simulink model "test"  (Simulink 7.4)
settings: Solver=ode45  StartTime=0.0  StopTime=100  MaxStep=0.05  RelTol=1e-3
values from neighbouring files (symbols this model uses):
  n_delay = [0; 40]    [setup.m]
  P_D = x(end)    [comp_rig_parallel_linearized.m]    (also in comp_rig_tank.m = x(1); get_tank_deriv.m = x(1); setup.m = xinit(end); test_linearization.m = P_D_init + delta_x(end,i))
  Ts = 0.05    [const_sim.m]
  uoff1 = [0.304, 0.405, 0.393, 0]'    [const_sim.m]
  uoff2 = [0.304, 0.405, 0.393, 0]'    [const_sim.m]
  xinit = [ 0.87171 1.0425 0.17319 400.38      0 0.98528 1.1784 0.17319 400.38      0 1.0116 ]    [setup.m]    (also in test_linearization.m = [0.890; 1.096; 0.159; 426; 0)
settings Model: Creator=chkajon  LastModifiedBy=chkajon

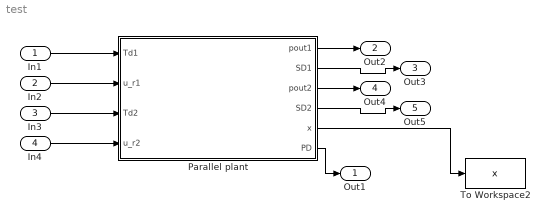
== system test ==
  In1 : Inport  OutDataType=fixdt(1, 16)  OutScaling=2^0
  In2 : Inport  Port=2  OutDataType=fixdt(1, 16)  OutScaling=2^0
  In3 : Inport  Port=3  OutDataType=fixdt(1, 16)  OutScaling=2^0
  In4 : Inport  Port=4  OutDataType=fixdt(1, 16)  OutScaling=2^0
  Parallel plant : Subsystem  mask{x_init_total=xinit, disturbances_on=off, disturbances_symm=off, dist_t_in=0, dist1_in=0, dist2_in=0}
      mask prompts: x_init_total "Initial state"; disturbances_on "Activate disturbances"; disturbances_symm "Symmetric disturbances"; dist_t_in "Disturbance times (up to 2)"; dist1_in "Disturbance 1 values (u1in, u1out, ud[, u2in, u2out])"; dist2_in "Disturbance 2 values"
      mask init:
      | dist1 = zeros(5,1);
      | dist2 = dist1;
      | dist_t = zeros(2,1);
      | 
      | if disturbances_on
      |     for i=1:min(5,length(dist1_in))
      |         dist1(i) = dist1_in(i);
      |     end
      |     for i=1:min(5,length(dist2_in))
      |         dist2(i) = dist2_in(i);
      |     end
      |     for i=1:min(2,length(dist_t_in))
      |         dist_t(i) = dist_t_in(i);
      |     end
      |     
      |     if disturbances_symm
      |         dist1(4) = dist1(1);
      |         dist1(5) = dist1(2);
      |         dist2(4) = dist2(1);
      |         dist2(5) = dist2(2);
      |     end
      | end
      | 
      | x_init1 = x_init_total(1:5);
      | x_init2 = x_init_total(6:10);
  To Workspace2 : ToWorkspace  VariableName=x  SampleTime=-1  SaveFormat=Structure With Time
  Out1 : Outport  OutDataType=fixdt(1, 16)  OutScaling=2^0
  Out2 : Outport  Port=2  OutDataType=fixdt(1, 16)  OutScaling=2^0
  Out3 : Outport  Port=3  OutDataType=fixdt(1, 16)  OutScaling=2^0
  Out4 : Outport  Port=4  OutDataType=fixdt(1, 16)  OutScaling=2^0
  Out5 : Outport  Port=5  OutDataType=fixdt(1, 16)  OutScaling=2^0
  wires:
  In1/1 -> Parallel plant/1(Td1)
  In2/1 -> Parallel plant/2(u_r1)
  In3/1 -> Parallel plant/3(Td2)
  In4/1 -> Parallel plant/4(u_r2)
  Parallel plant/5(x) -> To Workspace2/1
  Parallel plant/6(PD) -> Out1/1
  Parallel plant/1(pout1) -> Out2/1
  Parallel plant/2(SD1) -> Out3/1
  Parallel plant/3(pout2) -> Out4/1
  Parallel plant/4(SD2) -> Out5/1

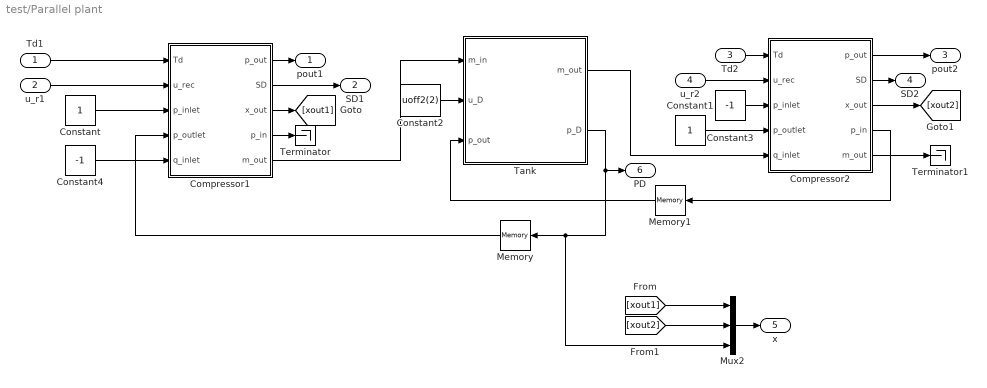
== system test/Parallel plant ==
  Td1 : Inport  OutDataType=fixdt(1, 16)  OutScaling=2^0
  u_r1 : Inport  Port=2  OutDataType=fixdt(1, 16)  OutScaling=2^0
  Td2 : Inport  Port=3  OutDataType=fixdt(1, 16)  OutScaling=2^0
  u_r2 : Inport  Port=4  OutDataType=fixdt(1, 16)  OutScaling=2^0
  Compressor1 : Subsystem  mask(Compressor){x_init=x_init1, Td_off=uoff1(1), u_in=uoff1(2), u_out=uoff1(3), u_rec=uoff1(4), t_delay=n_delay(2)*Ts, use_dist=on, u_out_dist=[dist1(1); dist2(1)], u_out_time=dist_t, u_in_dist=[dist1(2); dist2(2)], u_in_time=dist_t}
      mask prompts: x_init "Intial state"; Td_off "Torque offset"; u_in "Input valve setting"; u_out "Output valve setting"; u_rec "Recycle valve offset"; t_delay "Recycle valve time delay"; use_dist "Activate valve disturbances"; u_out_dist "Output valve disturbance magnitudes (up to 2)"; u_out_time "Output valve disturbance times (up to 2)"; u_in_dist "Input valve disturbance magnitudes (up to 2)"; u_in_time "Input valve disturbance times (up to 2)"
      mask help: Compressor with tunable inputs.
      mask init:
      | if use_dist
      |     n = min(length(u_out_dist),length(u_out_time));
      |     if n==0
      |         u_out_dist = [0;0];
      |         u_out_time = [0;0];
      |     elseif n==1
      |         u_out_dist = [u_out_dist(1);0];
      |         u_out_time = [u_out_time(1);0];
      |     else
      |         u_out_dist = [u_out_dist(1);u_out_dist(2)];
      |         u_out_time = [u_out_time(1); u_out_time(2)];
      |     end
      |     
      |     n = min(length(u_in_dist),length(u_in_time));
      |     if n==0
      |         u_in_dist = [0;0];
      |         u_in_time = [0;0];
      |     elseif n==1
      |         u_in_dist = [u_in_dist(1);0];
      |         u_in_time = [u_in_time(1);0];
      |     else
      |         u_in_dist = [u_in_dist(1);u_in_dist(2)];
      |         u_in_time = [u_in_time(1); u_in_time(2)];
      |     end
      | else
      |     u_out_dist = [0;0];
      |     u_out_time = [0;0];
      |     u_in_dist = [0;0];
      |     u_in_time = [0;0];
      | end
      mask TabNameString: Disturbances,Inputs,Inputs,Inputs,Inputs,Inputs,Disturbances,Disturbances,Disturbances,Disturbances,Disturbances
  Compressor2 : Subsystem  mask(Compressor){x_init=x_init2, Td_off=uoff2(1), u_in=uoff2(2), u_out=uoff2(3), u_rec=uoff2(4), t_delay=n_delay(2)*Ts, use_dist=on, u_out_dist=[dist1(4); dist2(4)], u_out_time=dist_t, u_in_dist=[dist1(5); dist2(5)], u_in_time=dist_t}
      mask prompts: x_init "Intial state"; Td_off "Torque offset"; u_in "Input valve setting"; u_out "Output valve setting"; u_rec "Recycle valve offset"; t_delay "Recycle valve time delay"; use_dist "Activate valve disturbances"; u_out_dist "Output valve disturbance magnitudes (up to 2)"; u_out_time "Output valve disturbance times (up to 2)"; u_in_dist "Input valve disturbance magnitudes (up to 2)"; u_in_time "Input valve disturbance times (up to 2)"
      mask help: Compressor with tunable inputs.
      mask init: same as test/Parallel plant/Compressor1
      mask TabNameString: Disturbances,Inputs,Inputs,Inputs,Inputs,Inputs,Disturbances,Disturbances,Disturbances,Disturbances,Disturbances
  Constant : Constant  OutDataType=fixdt(1, 16)  OutScaling=2^0
  Constant1 : Constant  OutDataType=fixdt(1, 16)  OutScaling=2^0
  Constant2 : Constant  Value=uoff2(2)  OutDataType=fixdt(1, 16)  OutScaling=2^0
  Constant3 : Constant  Value=-1  OutDataType=fixdt(1, 16)  OutScaling=2^0
  Constant4 : Constant  Value=-1  OutDataType=fixdt(1, 16)  OutScaling=2^0
  Memory : Memory  X0=P_D
  Memory1 : Memory  X0=x_init_total(6)
  Mux2 : Mux  Inputs=3
  Tank : Subsystem
  Terminator : Terminator
  Terminator1 : Terminator
  pout1 : Outport  OutDataType=fixdt(1, 16)  OutScaling=2^0
  SD1 : Outport  Port=2  OutDataType=fixdt(1, 16)  OutScaling=2^0
  pout2 : Outport  Port=3  OutDataType=fixdt(1, 16)  OutScaling=2^0
  SD2 : Outport  Port=4  OutDataType=fixdt(1, 16)  OutScaling=2^0
  x : Outport  Port=5  OutDataType=fixdt(1, 16)  OutScaling=2^0
  PD : Outport  Port=6  OutDataType=fixdt(1, 16)  OutScaling=2^0
  wires:
  Memory1/1 -> Tank/3(p_out)
  Compressor2/4(p_in) -> Memory1/1
  Constant2/1 -> Tank/2(u_D)
  Tank/1(m_out) -> Compressor2/5(q_inlet)
  Tank/2(p_D) -> PD/1, Memory/1, Mux2/3
  Compressor2/3(x_out) -> [xout2]
  Compressor2/2(SD) -> SD2/1
  Compressor2/1(p_out) -> pout2/1
  Compressor1/3(x_out) -> [xout1]
  Compressor1/2(SD) -> SD1/1
  Constant1/1 -> Compressor2/4(p_outlet)
  Compressor1/1(p_out) -> pout1/1
  Mux2/1 -> x/1
  [xout2] -> Mux2/2
  [xout1] -> Mux2/1
  u_r2/1 -> Compressor2/2(u_rec)
  Td2/1 -> Compressor2/1(Td)
  Constant3/1 -> Compressor2/3(p_inlet)
  Compressor1/5(m_out) -> Tank/1(m_in)
  Compressor1/4(p_in) -> Terminator/1
  Compressor2/5(m_out) -> Terminator1/1
  Memory/1 -> Compressor1/4(p_outlet)
  Td1/1 -> Compressor1/1(Td)
  u_r1/1 -> Compressor1/2(u_rec)
  Constant/1 -> Compressor1/3(p_inlet)
  Constant4/1 -> Compressor1/5(q_inlet)

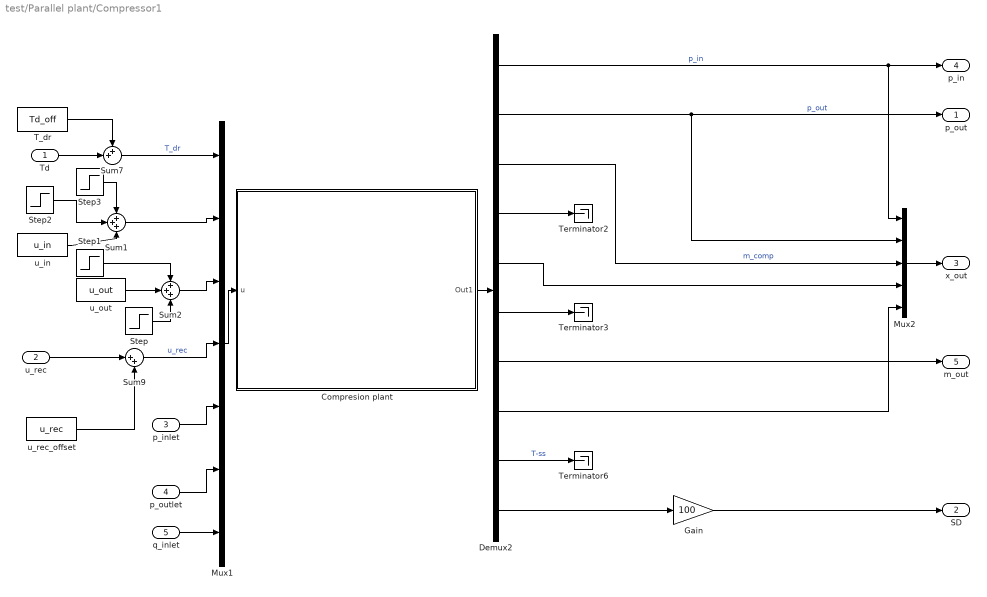
== system test/Parallel plant/Compressor1 ==
  Td : Inport  OutDataType=fixdt(1, 16)  OutScaling=2^0
  u_rec : Inport  Port=2  OutDataType=fixdt(1, 16)  OutScaling=2^0
  p_inlet : Inport  Port=3  OutDataType=fixdt(1, 16)  OutScaling=2^0
  p_outlet : Inport  Port=4  OutDataType=fixdt(1, 16)  OutScaling=2^0
  q_inlet : Inport  Port=5  OutDataType=fixdt(1, 16)  OutScaling=2^0
  Compresion plant : Subsystem
      mask Display: image(imread('comp_plant.jpg'))
  Demux2 : Demux  Outputs=10
  Gain : Gain  Gain=100  ParameterDataType=fixdt(1, 16)  ParameterScaling=2^0  OutDataType=fixdt(1, 16)  OutScaling=2^0
  Mux1 : Mux  Inputs=7
  Mux2 : Mux  Inputs=5
  Step : Step  Time=u_out_time(2)  After=u_out_dist(2)  SampleTime=0
  Step1 : Step  Time=u_out_time(1)  After=u_out_dist(1)  SampleTime=0
  Step2 : Step  Time=u_in_time(2)  After=u_in_dist(2)  SampleTime=0
  Step3 : Step  Time=u_in_time(1)  After=u_in_dist(1)  SampleTime=0
  Sum1 : Sum  Inputs=+++
  Sum2 : Sum  Inputs=+++
  Sum7 : Sum  Inputs=++|
  Sum9 : Sum  Inputs=|++
  T_dr : Constant  Value=Td_off
  Terminator2 : Terminator
  Terminator3 : Terminator
  Terminator6 : Terminator
  u_in : Constant  Value=u_in
  u_out : Constant  Value=u_out
  u_rec_offset : Constant  Value=u_rec
  p_out : Outport  OutDataType=fixdt(1, 16)  OutScaling=2^0
  SD : Outport  Port=2  OutDataType=fixdt(1, 16)  OutScaling=2^0
  x_out : Outport  Port=3  OutDataType=fixdt(1, 16)  OutScaling=2^0
  p_in : Outport  Port=4  OutDataType=fixdt(1, 16)  OutScaling=2^0
  m_out : Outport  Port=5  OutDataType=fixdt(1, 16)  OutScaling=2^0
  wires:
  Gain/1 -> SD/1
  q_inlet/1 -> Mux1/7
  Mux2/1 -> x_out/1
  Demux2/9 -> Terminator6/1  "T-ss"
  Sum2/1 -> Mux1/3
  Step/1 -> Sum2/3
  p_inlet/1 -> Mux1/5
  Demux2/10 -> Gain/1
  u_rec_offset/1 -> Sum9/2
  Demux2/5 -> Mux2/4
  Demux2/1 -> Mux2/1, p_in/1  "p_in"
  Demux2/2 -> p_out/1, Mux2/2  "p_out"
  Sum9/1 -> Mux1/4  "u_rec"
  Sum7/1 -> Mux1/1  "T_dr"
  u_rec/1 -> Sum9/1
  u_out/1 -> Sum2/2
  Demux2/7 -> m_out/1
  Demux2/8 -> Mux2/5
  Demux2/6 -> Terminator3/1
  Mux1/1 -> Compresion plant/1(u)
  Compresion plant/1(Out1) -> Demux2/1
  Step1/1 -> Sum2/1
  Demux2/3 -> Mux2/3  "m_comp"
  Demux2/4 -> Terminator2/1
  T_dr/1 -> Sum7/1
  Td/1 -> Sum7/2
  Step3/1 -> Sum1/1
  Step2/1 -> Sum1/2
  u_in/1 -> Sum1/3
  Sum1/1 -> Mux1/2
  p_outlet/1 -> Mux1/6

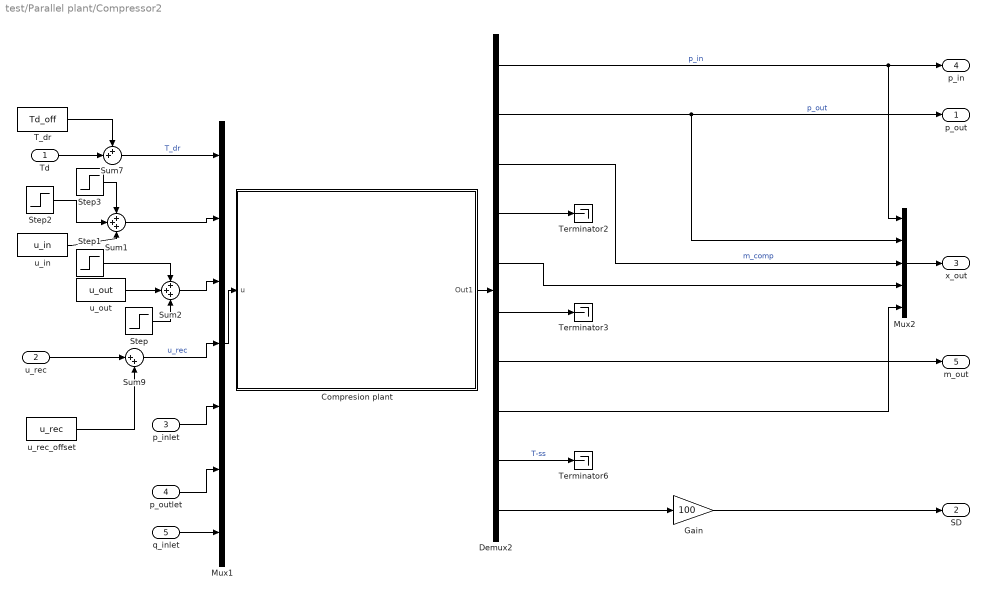
== system test/Parallel plant/Compressor2 ==
  Td : Inport  OutDataType=fixdt(1, 16)  OutScaling=2^0
  u_rec : Inport  Port=2  OutDataType=fixdt(1, 16)  OutScaling=2^0
  p_inlet : Inport  Port=3  OutDataType=fixdt(1, 16)  OutScaling=2^0
  p_outlet : Inport  Port=4  OutDataType=fixdt(1, 16)  OutScaling=2^0
  q_inlet : Inport  Port=5  OutDataType=fixdt(1, 16)  OutScaling=2^0
  Compresion plant : Subsystem
      mask Display: image(imread('comp_plant.jpg'))
  Demux2 : Demux  Outputs=10
  Gain : Gain  Gain=100  ParameterDataType=fixdt(1, 16)  ParameterScaling=2^0  OutDataType=fixdt(1, 16)  OutScaling=2^0
  Mux1 : Mux  Inputs=7
  Mux2 : Mux  Inputs=5
  Step : Step  Time=u_out_time(2)  After=u_out_dist(2)  SampleTime=0
  Step1 : Step  Time=u_out_time(1)  After=u_out_dist(1)  SampleTime=0
  Step2 : Step  Time=u_in_time(2)  After=u_in_dist(2)  SampleTime=0
  Step3 : Step  Time=u_in_time(1)  After=u_in_dist(1)  SampleTime=0
  Sum1 : Sum  Inputs=+++
  Sum2 : Sum  Inputs=+++
  Sum7 : Sum  Inputs=++|
  Sum9 : Sum  Inputs=|++
  T_dr : Constant  Value=Td_off
  Terminator2 : Terminator
  Terminator3 : Terminator
  Terminator6 : Terminator
  u_in : Constant  Value=u_in
  u_out : Constant  Value=u_out
  u_rec_offset : Constant  Value=u_rec
  p_out : Outport  OutDataType=fixdt(1, 16)  OutScaling=2^0
  SD : Outport  Port=2  OutDataType=fixdt(1, 16)  OutScaling=2^0
  x_out : Outport  Port=3  OutDataType=fixdt(1, 16)  OutScaling=2^0
  p_in : Outport  Port=4  OutDataType=fixdt(1, 16)  OutScaling=2^0
  m_out : Outport  Port=5  OutDataType=fixdt(1, 16)  OutScaling=2^0
  wires:
  Gain/1 -> SD/1
  q_inlet/1 -> Mux1/7
  Mux2/1 -> x_out/1
  Demux2/9 -> Terminator6/1  "T-ss"
  Sum2/1 -> Mux1/3
  Step/1 -> Sum2/3
  p_inlet/1 -> Mux1/5
  Demux2/10 -> Gain/1
  u_rec_offset/1 -> Sum9/2
  Demux2/5 -> Mux2/4
  Demux2/1 -> Mux2/1, p_in/1  "p_in"
  Demux2/2 -> p_out/1, Mux2/2  "p_out"
  Sum9/1 -> Mux1/4  "u_rec"
  Sum7/1 -> Mux1/1  "T_dr"
  u_rec/1 -> Sum9/1
  u_out/1 -> Sum2/2
  Demux2/7 -> m_out/1
  Demux2/8 -> Mux2/5
  Demux2/6 -> Terminator3/1
  Mux1/1 -> Compresion plant/1(u)
  Compresion plant/1(Out1) -> Demux2/1
  Step1/1 -> Sum2/1
  Demux2/3 -> Mux2/3  "m_comp"
  Demux2/4 -> Terminator2/1
  T_dr/1 -> Sum7/1
  Td/1 -> Sum7/2
  Step3/1 -> Sum1/1
  Step2/1 -> Sum1/2
  u_in/1 -> Sum1/3
  Sum1/1 -> Mux1/2
  p_outlet/1 -> Mux1/6

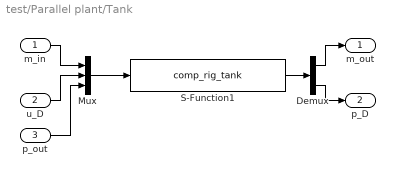
== system test/Parallel plant/Tank ==
  m_in : Inport  OutDataType=fixdt(1, 16)  OutScaling=2^0
  u_D : Inport  Port=2  OutDataType=fixdt(1, 16)  OutScaling=2^0
  p_out : Inport  Port=3  OutDataType=fixdt(1, 16)  OutScaling=2^0
  Demux : Demux  Outputs=2
  Mux : Mux  Inputs=3
  S-Function1 : S-Function  FunctionName=comp_rig_tank  Parameters=[], P_D  EnableBusSupport=off
  m_out : Outport  OutDataType=fixdt(1, 16)  OutScaling=2^0
  p_D : Outport  Port=2  OutDataType=fixdt(1, 16)  OutScaling=2^0
  wires:
  p_out/1 -> Mux/3
  S-Function1/1 -> Demux/1
  Demux/1 -> m_out/1
  Demux/2 -> p_D/1
  Mux/1 -> S-Function1/1
  m_in/1 -> Mux/1
  u_D/1 -> Mux/2

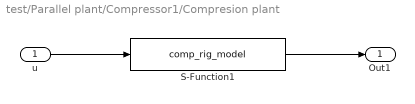
== system test/Parallel plant/Compressor1/Compresion plant ==
  u : Inport
  S-Function1 : S-Function  FunctionName=comp_rig_model  Parameters=[], x_init  EnableBusSupport=off
  Out1 : Outport
  wires:
  u/1 -> S-Function1/1
  S-Function1/1 -> Out1/1

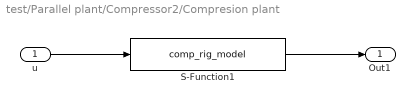
== system test/Parallel plant/Compressor2/Compresion plant ==
  u : Inport
  S-Function1 : S-Function  FunctionName=comp_rig_model  Parameters=[], x_init  EnableBusSupport=off
  Out1 : Outport
  wires:
  u/1 -> S-Function1/1
  S-Function1/1 -> Out1/1
